simulink model "BlockDiagram"  (R2024a)
settings: Solver=FixedStepAuto  StartTime=0.0  StopTime=Tsim  FixedStep=Tsim/(impulse_len - 1)  RelTol=1e-9
values from neighbouring files (symbols this model uses):
  C = 10e-6    (= 1e-05)    [Lab2.m]
  I0 = 1e-2    (= 0.01)    [Lab2.m]
  L = 0.2    [Lab2.m]
  N = 2    [Lab2.m]
  R = 100    [Lab2.m]
  V0 = 1    [Lab2.m]
settings Model: Creator=pablo  LastModifiedBy=pablo
settings DataIOCC: ReturnWorkspaceOutputs=off

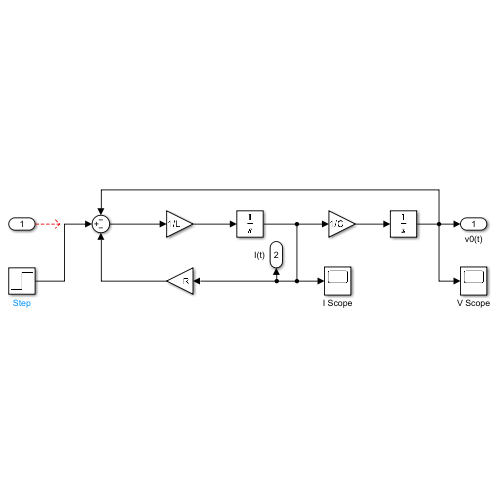
[thumbnail: Simulink's stored preview of the top-level diagram]
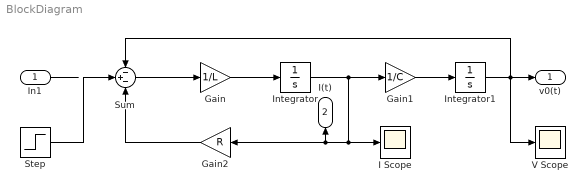
== system BlockDiagram ==
  In1 : Inport
  Gain : Gain  Gain=1/L
  Gain1 : Gain  Gain=1/C
  Gain2 : Gain  Gain=R
  I Scope : Scope
  Integrator : Integrator  InitialCondition=I0
  Integrator1 : Integrator  InitialCondition=V0
  Step : Step  Time=0  After=N  SampleTime=0
  Sum : Sum  Inputs=-+-
  V Scope : Scope
  v0(t) : Outport
  I(t) : Outport  Port=2
  wires:
  In1/1 -> ?
  Sum/1 -> Gain/1
  Gain/1 -> Integrator/1
  Integrator/1 -> I(t)/1, Gain2/1, I Scope/1, Gain1/1
  Gain1/1 -> Integrator1/1
  Gain2/1 -> Sum/3
  Integrator1/1 -> v0(t)/1, V Scope/1, Sum/1
  Step/1 -> Sum/2
